simulink model "ArujanHangingCrane"  (R2023b)
settings: Solver=VariableStepAuto  StartTime=0.0  StopTime=45  RelTol=1e-3
settings Model: Creator=admin  LastModifiedBy=admin

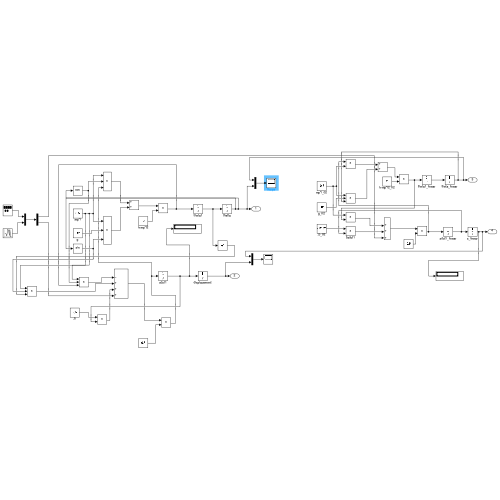
[thumbnail: Simulink's stored preview of the top-level diagram]
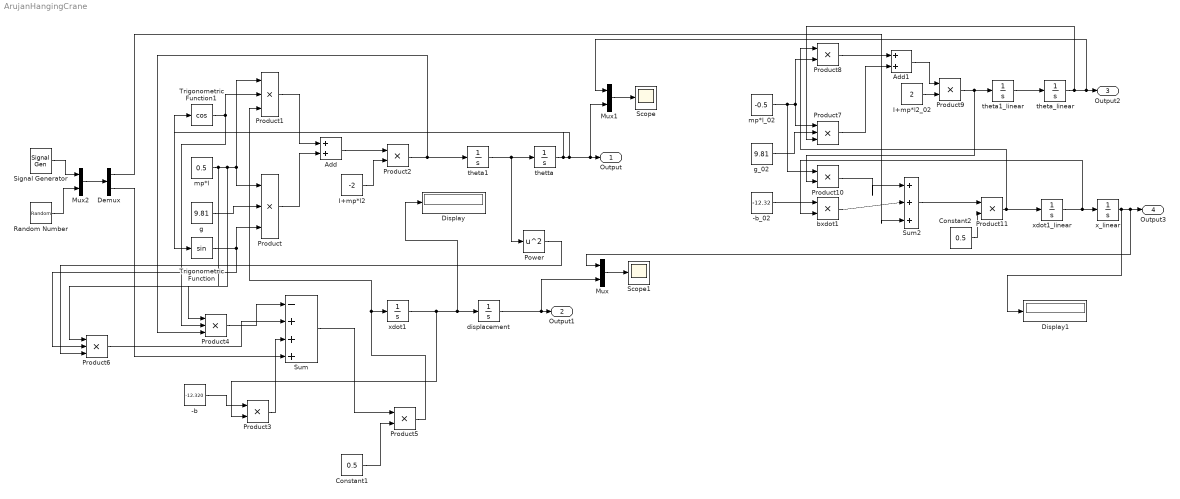
== system ArujanHangingCrane ==
  -b : Constant  Value=-12.320
  -b_02 : Constant  Value=-12.32
  Add : Sum
  Add1 : Sum
  Constant1 : Constant  Value=0.5
  Constant2 : Constant  Value=0.5
  Demux : Demux  Outputs=2
  Display : Display
  Display1 : Display
  I+mp*l2 : Constant  Value=-2
  I+mp*l2_02 : Constant  Value=2
  Mux : Mux  Inputs=2
  Mux1 : Mux  Inputs=2
  Mux2 : Mux  Inputs=2
  Power : Math  Operator=square
  Product{,1,4,6..7} (5 alike) : Product  Inputs=3
  Product{2..3,5,8..11} (7 alike) : Product
  Random Number : RandomNumber  SampleTime=0.1
  Scope : Scope
  Scope1 : Scope
  Signal Generator : SignalGenerator  Units=rad/sec
  Sum : Sum  Inputs=|-+++
  Sum2 : Sum  Inputs=|+++
  Trigonometric Function : Trigonometry
  Trigonometric Function1 : Trigonometry  Operator=cos
  bxdot1 : Product
  displacement : Integrator
  g : Constant  Value=9.81
  g_02 : Constant  Value=9.81
  mp*l : Constant  Value=0.5
  mp*l_02 : Constant  Value=-0.5
  theta1 : Integrator
  theta1_linear : Integrator
  theta_linear : Integrator
  thetta : Integrator
  x_linear : Integrator
  xdot1 : Integrator
  xdot1_linear : Integrator
  Output : Outport
  Output1 : Outport  Port=2
  Output2 : Outport  Port=3
  Output3 : Outport  Port=4
  wires:
  mp*l/1 -> Product6/1, Product4/1, Product1/1, Product/1
  g/1 -> Product/2
  Trigonometric Function/1 -> Product6/2, Product/3
  Product1/1 -> Add/1
  Product/1 -> Add/2
  Trigonometric Function1/1 -> Product4/2, Product1/2
  Add/1 -> Product2/1
  Product2/1 -> Product4/3, theta1/1
  theta1/1 -> Power/1, thetta/1
  thetta/1 -> Trigonometric Function1/1, Trigonometric Function/1, Mux1/2, Output/1
  I+mp*l2/1 -> Product2/2
  xdot1/1 -> Product3/2, Display/1, displacement/1
  displacement/1 -> Mux/2, Output1/1
  -b/1 -> Product3/1
  Product3/1 -> Sum/3
  Product4/1 -> Sum/1
  Power/1 -> Product6/3
  Product6/1 -> Sum/2
  Sum/1 -> Product5/1
  Constant1/1 -> Product5/2
  Product5/1 -> Product1/3, xdot1/1
  Random Number/1 -> Mux2/2
  mp*l_02/1 -> Product10/1, Product8/2, Product7/1
  g_02/1 -> Product7/2
  I+mp*l2_02/1 -> Product9/2
  Add1/1 -> Product9/1
  Product8/1 -> Add1/1
  Product7/1 -> Add1/2
  Product9/1 -> Product10/2, theta1_linear/1
  theta1_linear/1 -> theta_linear/1
  theta_linear/1 -> Product7/3, Mux1/1, Output2/1
  -b_02/1 -> bxdot1/1
  Product10/1 -> Sum2/1
  bxdot1/1 -> Sum2/2
  Mux2/1 -> Demux/1
  Demux/2 -> Sum/4
  Demux/1 -> Sum2/3
  Sum2/1 -> Product11/1
  Constant2/1 -> Product11/2
  Product11/1 -> Product8/1, xdot1_linear/1
  xdot1_linear/1 -> bxdot1/2, x_linear/1
  x_linear/1 -> Display1/1, Mux/1, Output3/1
  Mux1/1 -> Scope/1
  Mux/1 -> Scope1/1
  Signal Generator/1 -> Mux2/1
